simulink model "Speed_fuzzy"  (Simulink 8.1)
settings: Solver=ode23tb  StartTime=0.0  StopTime=4  RelTol=1e-3
InitFcn:
  | ts=100e-6;
StartFcn:
  | close all
libraries: powerlib_extras x1, fuzblock x1, simulink x1
CloseFcn:
  | close all
settings Model: Creator=srikanth  LastModifiedBy=LALIT
settings DataIOCC: LimitDataPoints=off  SaveOutput=off  SaveTime=off  TimeSaveName=t  OutputSaveName=speed,torque,ref
settings DebuggingCC: SolverPrmCheckMsg=none
settings GRTTargetCC: CodeReplacementLibrary=C89/C90 (ANSI)

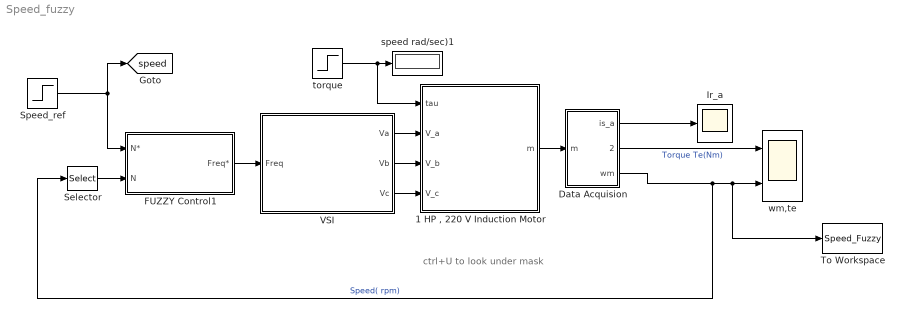
== system Speed_fuzzy ==
  note: ctrl+U to look under mask
  "1 HP , 220 V Induction Motor" : Subsystem  mask(Induction Motor: By SRIKANTH D){Rs=10.1, Ls=(15.81+245.8954)/(2*pi*50), Rr=9.8546, Lr=(15.81+245.8954)/(2*pi*50), Lm=(245.8954)/(2*pi*50), J=0.0088, P=4}
      mask prompts: Rs "Stator Resistance  Rs [ohms] :"; Ls "Stator Inductance Ls [Hendry] :"; Rr "Rotor Resistance Rr [ohms] :"; Lr "Rotor Inductance Lr [Hendry] :"; Lm "Mutual Inductance Lm [Hendry] :"; J "Rotor Inertia J [Kg-m2] :"; P "Number of Poles p :"
      mask help: Dynamic Modelling of Induction by using Mathematic Equations
      mask Display: fprintf('Induction\nMotor')
  Data Acquision : Subsystem
  FUZZY Control1 : Subsystem
      mask Display: fprintf('PI\Control')
  Ir_a : Scope
      settings: TimeRange=2  YMin=-3  YMax=3  SampleTime=ts
  Selector : Selector  InputPortWidth=2  IndexOptions=Index vector (dialog)  Indices=[1]  OutputSizes=1
  Speed_ref : Step  Time=2  Before=500  After=1400  SampleTime=0
  To Workspace : ToWorkspace  VariableName=Speed_Fuzzy  SampleTime=-1  SaveFormat=Timeseries
  VSI : Subsystem
      mask init:
      | Vdc=220;
      mask Display: fprintf('Vdc = 220 V ')
  speed rad/sec)1 : Display
  torque : Step  SampleTime=0
  wm,te : Scope  NumInputPorts=2
      settings: TimeRange=4  YMin=0.5~450  YMax=3.75~1400  SampleInput=on  SampleTime=ts
  tag scope: speed=global
  wires:
  torque/1 -> speed rad/sec)1/1, "1 HP , 220 V Induction Motor"/1(tau)
  VSI/1(Va) -> "1 HP , 220 V Induction Motor"/2(V_a)
  VSI/2(Vb) -> "1 HP , 220 V Induction Motor"/3(V_b)
  VSI/3(Vc) -> "1 HP , 220 V Induction Motor"/4(V_c)
  "1 HP , 220 V Induction Motor"/1(m) -> Data Acquision/1(m)
  Data Acquision/3(wm) -> To Workspace/1, wm,te/2, Selector/1  "Speed( rpm)"
  Data Acquision/2(Te(Nm)) -> wm,te/1  "Torque Te(Nm)"
  Data Acquision/1(is_a) -> Ir_a/1
  Speed_ref/1 -> FUZZY Control1/1(N*), [speed]
  Selector/1 -> FUZZY Control1/2(N)
  FUZZY Control1/1(Freq*) -> VSI/1(Freq)

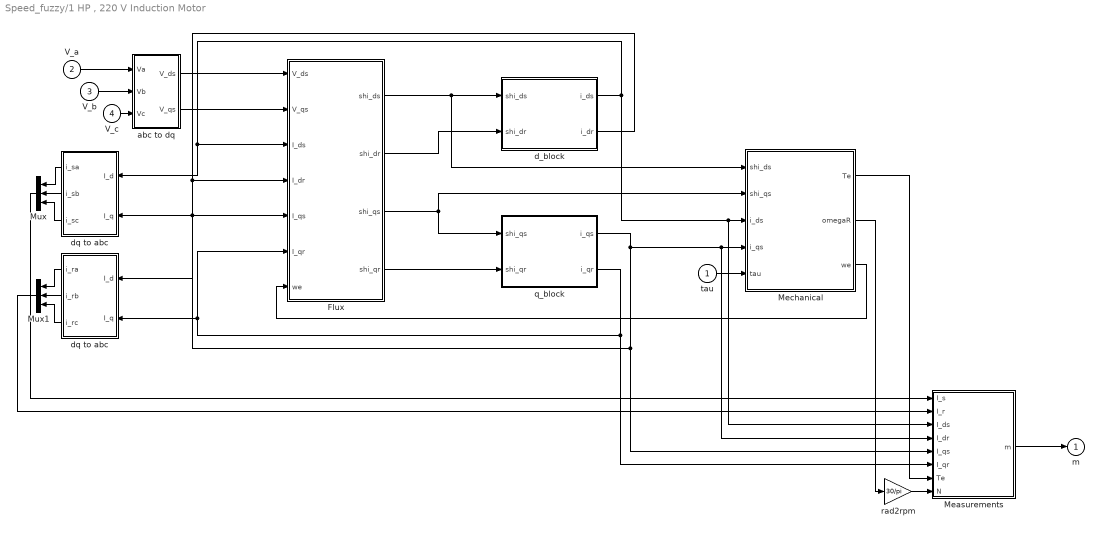
== system Speed_fuzzy/1 HP , 220 V Induction Motor ==
  tau : Inport
  V_a : Inport  Port=2
  V_b : Inport  Port=3
  V_c : Inport  Port=4
  Flux : Subsystem
  Measurements : Subsystem
  Mechanical : Subsystem
  Mux : Mux  Inputs=3
  Mux1 : Mux  Inputs=3
  abc to dq : Subsystem
  d_block : Subsystem
  dq to abc : Subsystem
  "dq to abc " : Subsystem
  q_block : Subsystem
  rad2rpm : Gain  Gain=30/pi
  m : Outport
  wires:
  Mechanical/2(omegaR) -> rad2rpm/1
  Mechanical/3(we) -> Flux/7(we)
  Flux/1(shi_ds) -> d_block/1(shi_ds), Mechanical/1(shi_ds)
  Flux/4("shi_qr ") -> q_block/2(shi_qr)
  d_block/1(i_ds) -> Mechanical/3(i_ds), Measurements/3(I_ds), dq to abc/1(I_d), Flux/3(I_ds)
  d_block/2(i_dr) -> Flux/4(I_dr), "dq to abc "/1(I_d)
  q_block/2(i_qr) -> Measurements/6(I_qr), "dq to abc "/2(I_q), Flux/6(I_qr)
  q_block/1(i_qs) -> Mechanical/4(i_qs), Measurements/4(I_dr), Measurements/5(I_qs), dq to abc/2(I_q), Flux/5(I_qs)
  Mechanical/1(Te) -> Measurements/7(Te)
  tau/1 -> Mechanical/5(tau)
  Flux/2("shi_dr ") -> d_block/2(shi_dr)
  Flux/3(shi_qs) -> q_block/1(shi_qs), Mechanical/2(shi_qs)
  abc to dq/1(V_ds) -> Flux/1(V_ds)
  abc to dq/2(V_qs) -> Flux/2(V_qs)
  V_c/1 -> abc to dq/3(Vc)
  V_b/1 -> abc to dq/2(Vb)
  V_a/1 -> abc to dq/1(Va)
  dq to abc/1(i_sa) -> Mux/1
  "dq to abc "/1(i_ra) -> Mux1/1
  dq to abc/2(i_sb) -> Mux/2
  dq to abc/3(i_sc) -> Mux/3
  "dq to abc "/3(i_rc) -> Mux1/3
  "dq to abc "/2(i_rb) -> Mux1/2
  Mux/1 -> Measurements/1(I_s)
  Mux1/1 -> Measurements/2(I_r)
  rad2rpm/1 -> Measurements/8(N)
  Measurements/1(m) -> m/1

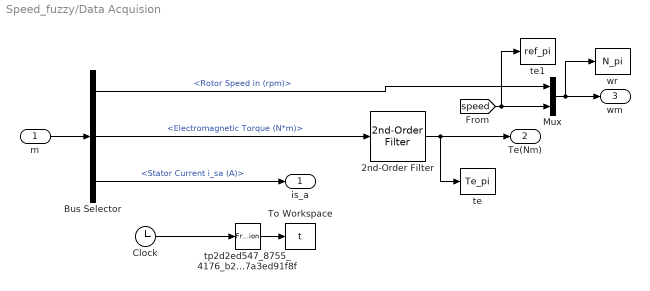
== system Speed_fuzzy/Data Acquision ==
  m : Inport
  2nd-Order Filter : powerlib_extras/Control  Blocks/2nd-Order Filter  FilterType=Lowpass  Fo=120  Zeta=0.707  Initialize=off  Vac_Init=[1 45 60]  Vdc_Init=-0.5  PlotResponse=off  param1=[1 500 1]
  Bus Selector : BusSelector  OutputSignals=Mechanical.Rotor Speed in (rpm),Mechanical.Electromagnetic Torque (N*m),Stator Measurement.Stator Current i_sa (A)
  Clock : Clock
  Mux : Mux  Inputs=2
  To Workspace : ToWorkspace  VariableName=t  SampleTime=ts
  te : ToWorkspace  VariableName=Te_pi  SampleTime=ts
  te1 : ToWorkspace  VariableName=ref_pi  SampleTime=ts
  tp2d2ed547_8755_4176_b2df_b47a3ed91f8f : FrameConversion  OutFrame=Sample-based
  wr : ToWorkspace  VariableName=N_pi  SampleTime=ts
  is_a : Outport
  Te(Nm) : Outport  Port=2
  wm : Outport  Port=3
  wires:
  2nd-Order Filter/1 -> Te(Nm)/1, te/1
  Bus Selector/2 -> 2nd-Order Filter/1  "<Electromagnetic Torque (N*m)>"
  m/1 -> Bus Selector/1
  Bus Selector/1 -> Mux/1  "<Rotor Speed in (rpm)>"
  Bus Selector/3 -> is_a/1  "<Stator Current i_sa (A)>"
  [speed] -> te1/1, Mux/2
  Mux/1 -> wm/1, wr/1
  Clock/1 -> tp2d2ed547_8755_4176_b2df_b47a3ed91f8f/1
  tp2d2ed547_8755_4176_b2df_b47a3ed91f8f/1 -> To Workspace/1

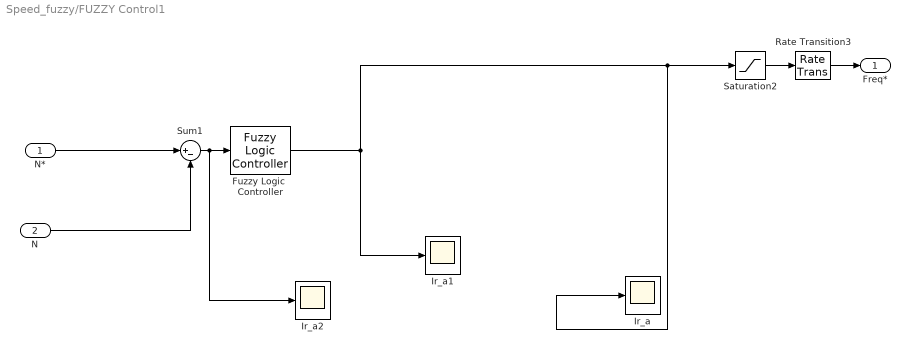
== system Speed_fuzzy/FUZZY Control1 ==
  N* : Inport
  N : Inport  Port=2
  Fuzzy Logic  Controller : fuzblock/Fuzzy Logic  Controller  fis=PMSG
  Ir_a : Scope
      settings: TimeRange=2  YMin=26.475  YMax=26.825  SaveName=ScopeData3  SampleTime=ts
  Ir_a1 : Scope
      settings: TimeRange=2  YMin=-3  YMax=3  SaveName=ScopeData4  SampleTime=ts
  Ir_a2 : Scope
      settings: TimeRange=2  YMin=1450  YMax=2150  SaveName=ScopeData5  SampleTime=ts
  Rate Transition3 : RateTransition  OutPortSampleTimeOpt=Inherit
  Saturation2 : Saturate  UpperLimit=50  LowerLimit=-50
  Sum1 : Sum  Inputs=|+-  SaturateOnIntegerOverflow=on  InputSameDT=on  OutDataTypeStr=Inherit: Same as first input
  Freq* : Outport
  wires:
  Sum1/1 -> Ir_a2/1, Fuzzy Logic  Controller/1
  N*/1 -> Sum1/1
  N/1 -> Sum1/2
  Saturation2/1 -> Rate Transition3/1
  Rate Transition3/1 -> Freq*/1
  Fuzzy Logic  Controller/1 -> Ir_a/1, Saturation2/1, Ir_a1/1

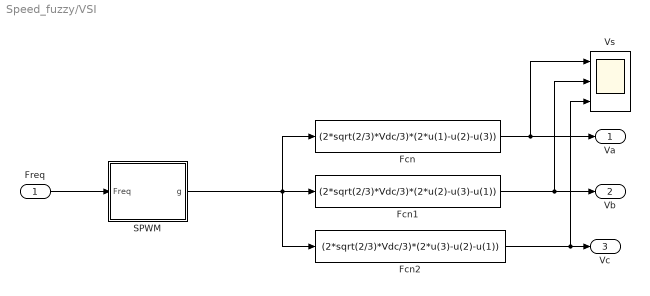
== system Speed_fuzzy/VSI ==
  Freq : Inport
  Fcn : Fcn  Expr=(2*sqrt(2/3)*Vdc/3)*(2*u(1)-u(2)-u(3))
  Fcn1 : Fcn  Expr=(2*sqrt(2/3)*Vdc/3)*(2*u(2)-u(3)-u(1))
  Fcn2 : Fcn  Expr=(2*sqrt(2/3)*Vdc/3)*(2*u(3)-u(2)-u(1))
  SPWM : Subsystem
  Vs : Scope  NumInputPorts=3
      settings: TimeRange=0.1701392689898436  YMin=-500~-500~-500  YMax=500~500~500  SaveName=voltage  SampleInput=on  SampleTime=ts
  Va : Outport
  Vb : Outport  Port=2
  Vc : Outport  Port=3
  wires:
  SPWM/1(g) -> Fcn2/1, Fcn/1, Fcn1/1
  Fcn1/1 -> Vb/1, Vs/2
  Fcn2/1 -> Vc/1, Vs/3
  Fcn/1 -> Va/1, Vs/1
  Freq/1 -> SPWM/1(Freq)

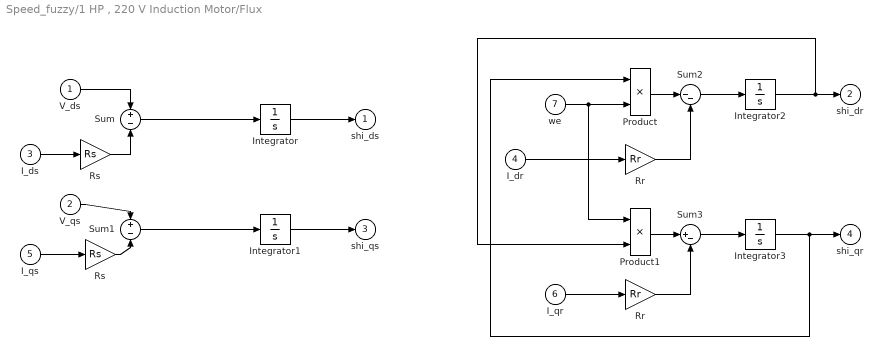
== system Speed_fuzzy/1 HP , 220 V Induction Motor/Flux ==
  V_ds : Inport
  V_qs : Inport  Port=2
  I_ds : Inport  Port=3
  I_dr : Inport  Port=4
  I_qs : Inport  Port=5
  I_qr : Inport  Port=6
  we : Inport  Port=7
  Integrator{,1..3} (4 alike) : Integrator
  Product : Product
  Product1 : Product
  Rr : Gain  Gain=Rr
  "Rr " : Gain  Gain=Rr
  Rs : Gain  Gain=Rs
  "Rs " : Gain  Gain=Rs
  Sum : Sum  Inputs=+|-
  Sum1 : Sum  Inputs=+|-
  Sum2 : Sum  Inputs=|--
  Sum3 : Sum  Inputs=|+-
  shi_ds : Outport
  "shi_dr " : Outport  Port=2
  shi_qs : Outport  Port=3
  "shi_qr " : Outport  Port=4
  wires:
  Sum3/1 -> Integrator3/1
  "Rr "/1 -> Sum3/2
  Product1/1 -> Sum3/1
  I_qr/1 -> "Rr "/1
  Integrator2/1 -> "shi_dr "/1, Product1/2
  Sum2/1 -> Integrator2/1
  Product/1 -> Sum2/1
  Rr/1 -> Sum2/2
  I_dr/1 -> Rr/1
  Integrator3/1 -> "shi_qr "/1, Product/1
  we/1 -> Product1/1, Product/2
  "Rs "/1 -> Sum1/2
  Rs/1 -> Sum/2
  Integrator1/1 -> shi_qs/1
  Integrator/1 -> shi_ds/1
  Sum1/1 -> Integrator1/1
  V_qs/1 -> Sum1/1
  I_qs/1 -> "Rs "/1
  Sum/1 -> Integrator/1
  V_ds/1 -> Sum/1
  I_ds/1 -> Rs/1

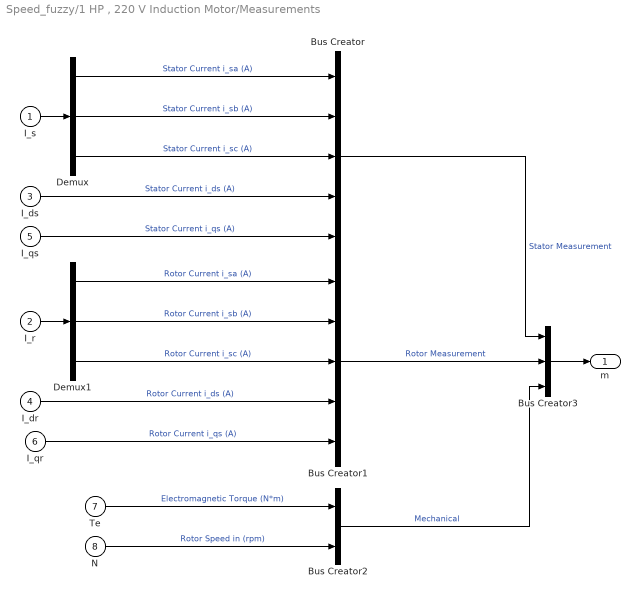
== system Speed_fuzzy/1 HP , 220 V Induction Motor/Measurements ==
  I_s : Inport
  I_r : Inport  Port=2
  I_ds : Inport  Port=3
  I_dr : Inport  Port=4
  I_qs : Inport  Port=5
  I_qr : Inport  Port=6
  Te : Inport  Port=7
  N : Inport  Port=8
  Bus Creator : BusCreator  Inputs=5
  Bus Creator1 : BusCreator  Inputs=5
  Bus Creator2 : BusCreator  Inputs=2
  Bus Creator3 : BusCreator  Inputs=3
  Demux : Demux  Outputs=3
  Demux1 : Demux  Outputs=3
  m : Outport
  wires:
  Bus Creator3/1 -> m/1
  Bus Creator2/1 -> Bus Creator3/3  "Mechanical"
  Bus Creator1/1 -> Bus Creator3/2  "Rotor Measurement"
  Bus Creator/1 -> Bus Creator3/1  "Stator Measurement"
  N/1 -> Bus Creator2/2  "Rotor Speed in (rpm)"
  Te/1 -> Bus Creator2/1  "Electromagnetic Torque (N*m)"
  I_qr/1 -> Bus Creator1/5  "Rotor Current i_qs (A)"
  I_dr/1 -> Bus Creator1/4  "Rotor Current i_ds (A)"
  Demux1/3 -> Bus Creator1/3  "Rotor Current i_sc (A)"
  Demux1/2 -> Bus Creator1/2  "Rotor Current i_sb (A)"
  Demux1/1 -> Bus Creator1/1  "Rotor Current i_sa (A)"
  I_r/1 -> Demux1/1
  I_qs/1 -> Bus Creator/5  "Stator Current i_qs (A)"
  I_ds/1 -> Bus Creator/4  "Stator Current i_ds (A)"
  Demux/3 -> Bus Creator/3  "Stator Current i_sc (A)"
  Demux/2 -> Bus Creator/2  "Stator Current i_sb (A)"
  Demux/1 -> Bus Creator/1  "Stator Current i_sa (A)"
  I_s/1 -> Demux/1

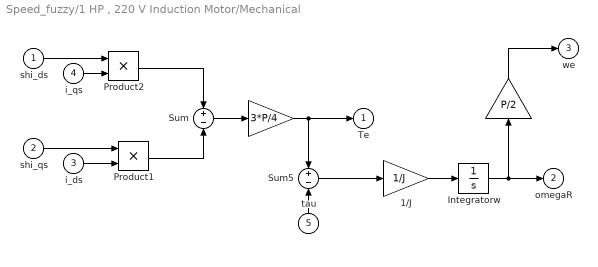
== system Speed_fuzzy/1 HP , 220 V Induction Motor/Mechanical ==
  shi_ds : Inport
  shi_qs : Inport  Port=2
  i_ds : Inport  Port=3
  i_qs : Inport  Port=4
  tau : Inport  Port=5
  " " : Gain  Gain=P/2  SaturateOnIntegerOverflow=on  OutDataTypeStr=Inherit: Same as input  ParamDataTypeStr=Inherit: Same as input
  "  " : Gain  Gain=3*P/4  SaturateOnIntegerOverflow=on  OutDataTypeStr=Inherit: Same as input  ParamDataTypeStr=Inherit: Same as input
  1/J : Gain  Gain=1/J  SaturateOnIntegerOverflow=on  OutDataTypeStr=Inherit: Same as input  ParamDataTypeStr=Inherit: Same as input
  Integratorw : Integrator
  Product1 : Product
  Product2 : Product
  Sum : Sum  Inputs=+|-
  Sum5 : Sum  Inputs=+-  SaturateOnIntegerOverflow=on  InputSameDT=on  OutDataTypeStr=Inherit: Same as first input
  Te : Outport
  omegaR : Outport  Port=2
  we : Outport  Port=3
  wires:
  " "/1 -> we/1
  Integratorw/1 -> omegaR/1, " "/1
  1/J/1 -> Integratorw/1
  Sum5/1 -> 1/J/1
  tau/1 -> Sum5/2
  "  "/1 -> Sum5/1, Te/1
  Sum/1 -> "  "/1
  Product2/1 -> Sum/1
  Product1/1 -> Sum/2
  i_ds/1 -> Product1/2
  shi_qs/1 -> Product1/1
  i_qs/1 -> Product2/2
  shi_ds/1 -> Product2/1

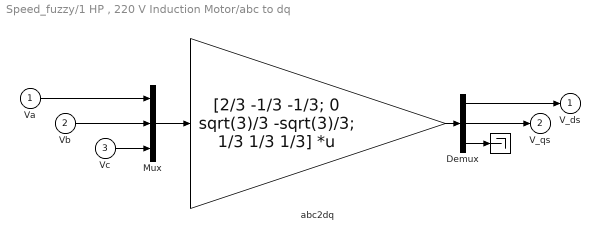
== system Speed_fuzzy/1 HP , 220 V Induction Motor/abc to dq ==
  Va : Inport
  Vb : Inport  Port=2
  Vc : Inport  Port=3
  "            " : Terminator
  Demux : Demux  Outputs=3
  Mux : Mux  Inputs=3
  abc2dq : Gain  Gain=[2/3 -1/3 -1/3; 0 sqrt(3)/3 -sqrt(3)/3; 1/3 1/3 1/3]  Multiplication=Matrix(K*u)  SaturateOnIntegerOverflow=on  OutDataTypeStr=Inherit: Same as input  ParamDataTypeStr=Inherit: Same as input
  V_ds : Outport
  V_qs : Outport  Port=2
  wires:
  Mux/1 -> abc2dq/1
  abc2dq/1 -> Demux/1
  Demux/2 -> V_qs/1
  Demux/1 -> V_ds/1
  Va/1 -> Mux/1
  Vb/1 -> Mux/2
  Vc/1 -> Mux/3
  Demux/3 -> "            "/1

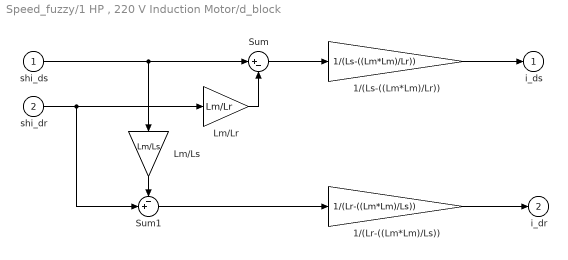
== system Speed_fuzzy/1 HP , 220 V Induction Motor/d_block ==
  shi_ds : Inport
  shi_dr : Inport  Port=2
  1/(Lr-((Lm*Lm)/Ls)) : Gain  Gain=1/(Lr-((Lm*Lm)/Ls))  SaturateOnIntegerOverflow=on  OutDataTypeStr=Inherit: Same as input  ParamDataTypeStr=Inherit: Same as input
  1/(Ls-((Lm*Lm)/Lr)) : Gain  Gain=1/(Ls-((Lm*Lm)/Lr))  SaturateOnIntegerOverflow=on  OutDataTypeStr=Inherit: Same as input  ParamDataTypeStr=Inherit: Same as input
  Lm/Lr : Gain  Gain=Lm/Lr
  Lm/Ls : Gain  Gain=Lm/Ls
  Sum : Sum  Inputs=|+-
  Sum1 : Sum  Inputs=-+|
  i_ds : Outport
  i_dr : Outport  Port=2
  wires:
  Sum1/1 -> 1/(Lr-((Lm*Lm)/Ls))/1
  Lm/Ls/1 -> Sum1/1
  Sum/1 -> 1/(Ls-((Lm*Lm)/Lr))/1
  Lm/Lr/1 -> Sum/2
  shi_dr/1 -> Sum1/2, Lm/Lr/1
  shi_ds/1 -> Lm/Ls/1, Sum/1
  1/(Lr-((Lm*Lm)/Ls))/1 -> i_dr/1
  1/(Ls-((Lm*Lm)/Lr))/1 -> i_ds/1

== system Speed_fuzzy/1 HP , 220 V Induction Motor/dq to abc ==
  I_d : Inport
  I_q : Inport  Port=2
  Demux : Demux  Outputs=3
  Gain : Gain  Gain=2/3  SaturateOnIntegerOverflow=on  OutDataTypeStr=Inherit: Same as input  ParamDataTypeStr=Inherit: Same as input
  Matrix Gain : Gain  Gain=[1 0;-0.5 -sqrt(3)/2;-0.5 sqrt(3)/2]  Multiplication=Matrix(K*u)  SaturateOnIntegerOverflow=on  OutDataTypeStr=Inherit: Same as input  ParamDataTypeStr=Inherit: Same as input
  Mux : Mux  Inputs=2
  i_sa : Outport
  i_sb : Outport  Port=2
  i_sc : Outport  Port=3
  wires:
  Demux/1 -> i_sa/1
  Demux/3 -> i_sc/1
  I_q/1 -> Mux/2
  I_d/1 -> Mux/1
  Demux/2 -> i_sb/1
  Matrix Gain/1 -> Gain/1
  Gain/1 -> Demux/1
  Mux/1 -> Matrix Gain/1

== system Speed_fuzzy/1 HP , 220 V Induction Motor/dq to abc  ==
  I_d : Inport
  I_q : Inport  Port=2
  Demux : Demux  Outputs=3
  Gain : Gain  Gain=2/3  SaturateOnIntegerOverflow=on  OutDataTypeStr=Inherit: Same as input  ParamDataTypeStr=Inherit: Same as input
  Matrix Gain : Gain  Gain=[1 0;-0.5 -sqrt(3)/2;-0.5 sqrt(3)/2]  Multiplication=Matrix(K*u)  SaturateOnIntegerOverflow=on  OutDataTypeStr=Inherit: Same as input  ParamDataTypeStr=Inherit: Same as input
  Mux : Mux  Inputs=2
  i_ra : Outport
  i_rb : Outport  Port=2
  i_rc : Outport  Port=3
  wires:
  Mux/1 -> Matrix Gain/1
  Gain/1 -> Demux/1
  Matrix Gain/1 -> Gain/1
  Demux/2 -> i_rb/1
  I_d/1 -> Mux/1
  I_q/1 -> Mux/2
  Demux/3 -> i_rc/1
  Demux/1 -> i_ra/1

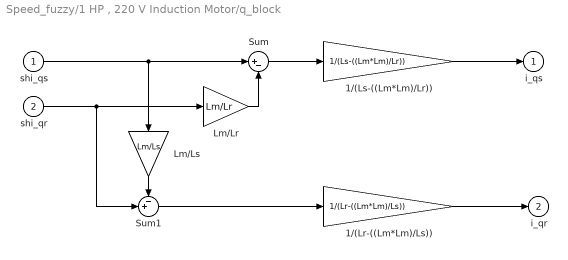
== system Speed_fuzzy/1 HP , 220 V Induction Motor/q_block ==
  shi_qs : Inport
  shi_qr : Inport  Port=2
  1/(Lr-((Lm*Lm)/Ls)) : Gain  Gain=1/(Lr-((Lm*Lm)/Ls))  SaturateOnIntegerOverflow=on  OutDataTypeStr=Inherit: Same as input  ParamDataTypeStr=Inherit: Same as input
  1/(Ls-((Lm*Lm)/Lr)) : Gain  Gain=1/(Ls-((Lm*Lm)/Lr))  SaturateOnIntegerOverflow=on  OutDataTypeStr=Inherit: Same as input  ParamDataTypeStr=Inherit: Same as input
  Lm/Lr : Gain  Gain=Lm/Lr
  Lm/Ls : Gain  Gain=Lm/Ls
  Sum : Sum  Inputs=|+-
  Sum1 : Sum  Inputs=-+|
  i_qs : Outport
  i_qr : Outport  Port=2
  wires:
  Sum1/1 -> 1/(Lr-((Lm*Lm)/Ls))/1
  Lm/Ls/1 -> Sum1/1
  Sum/1 -> 1/(Ls-((Lm*Lm)/Lr))/1
  Lm/Lr/1 -> Sum/2
  shi_qr/1 -> Lm/Lr/1, Sum1/2
  shi_qs/1 -> Lm/Ls/1, Sum/1
  1/(Lr-((Lm*Lm)/Ls))/1 -> i_qr/1
  1/(Ls-((Lm*Lm)/Lr))/1 -> i_qs/1

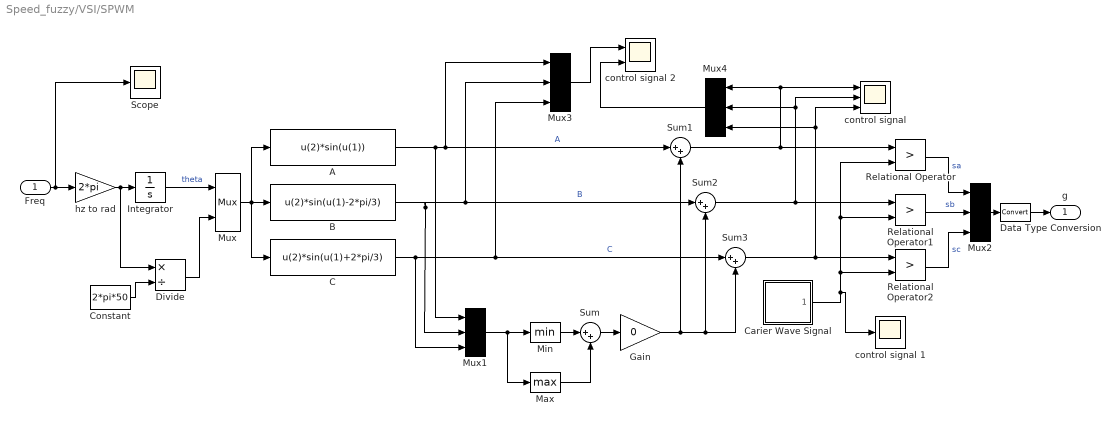
== system Speed_fuzzy/VSI/SPWM ==
  Freq : Inport
  A : Fcn  Expr=u(2)*sin(u(1))
  B : Fcn  Expr=u(2)*sin(u(1)-2*pi/3)
  C : Fcn  Expr=u(2)*sin(u(1)+2*pi/3)
  Carier Wave Signal : Subsystem  mask(Carrier Wave Generator:){A=1, fc=500}
      mask prompts: A "Amplitude"; fc "Carrier Wave Frequency"
      mask Display: fprintf('Carrier\nWave')
  Constant : Constant  Value=2*pi*50
  Data Type Conversion : DataTypeConversion
  Divide : Product  Inputs=*/
  Gain : Gain  Gain=0
  Integrator : Integrator
  Max : MinMax  Function=max
  Min : MinMax
  Mux : Mux  Inputs=2
      settings: DisplayOption=signals
  Mux{1..4} (4 alike) : Mux  Inputs=3
      settings: DisplayOption=signals
  Relational Operator : RelationalOperator  Operator=>  OutDataTypeStr=boolean
  Relational Operator1 : RelationalOperator  Operator=>  OutDataTypeStr=boolean
  Relational Operator2 : RelationalOperator  Operator=>  OutDataTypeStr=boolean
  Scope : Scope
      settings: TimeRange=3  YMin=30  YMax=50  SaveName=ScopeData2
  Sum{,1..3} (4 alike) : Sum  Inputs=|++
  "control signal " : Scope  NumInputPorts=3
      settings: TimeRange=0.5  YMin=-1.5~-1.5~-1.5  YMax=1.5~1.5~1.5
  control signal 1 : Scope
      settings: TimeRange=0.0117840461100045  YMin=-1  YMax=1  SampleTime=Ts
  control signal 2 : Scope  NumInputPorts=2
      settings: TimeRange=4  YMin=-1.5~-1.5  YMax=1.5~1.5  SaveName=ScopeData6
  hz to rad : Gain  Gain=2*pi
  g : Outport
  wires:
  Mux4/1 -> control signal 2/2
  Mux3/1 -> control signal 2/1
  Constant/1 -> Divide/2
  Divide/1 -> Mux/2
  Gain/1 -> Sum1/2, Sum3/2, Sum2/2
  Freq/1 -> hz to rad/1, Scope/1
  C/1 -> Mux3/3, Sum3/1, Mux1/3  "C"
  Mux/1 -> C/1, A/1, B/1
  Integrator/1 -> Mux/1  "theta"
  A/1 -> Mux3/1, Sum1/1, Mux1/1  "A"
  hz to rad/1 -> Divide/1, Integrator/1
  B/1 -> Mux3/2, Sum2/1, Mux1/2  "B"
  Min/1 -> Sum/1
  Max/1 -> Sum/2
  Carier Wave Signal/1("Carier Wave ") -> control signal 1/1, Relational Operator2/2, Relational Operator1/2, Relational Operator/2
  Relational Operator2/1 -> Mux2/3  "sc"
  Relational Operator1/1 -> Mux2/2  "sb"
  Relational Operator/1 -> Mux2/1  "sa"
  Mux1/1 -> Max/1, Min/1
  Sum/1 -> Gain/1
  Sum1/1 -> Mux4/1, "control signal "/1, Relational Operator/1
  Sum2/1 -> Mux4/2, "control signal "/2, Relational Operator1/1
  Sum3/1 -> Mux4/3, "control signal "/3, Relational Operator2/1
  Mux2/1 -> Data Type Conversion/1
  Data Type Conversion/1 -> g/1

== system Speed_fuzzy/VSI/SPWM/Carier Wave Signal ==
  Carier Wave : simulink/Sources/Repeating Sequence  rep_seq_t=[0 0.25 0.5 0.75 1]./fc  rep_seq_y=[0 1 0 -1 0].*A
  "Carier Wave " : Outport
  wires:
  Carier Wave/1 -> "Carier Wave "/1  "0 delay"
